simulink model "ofdm_rx"  (R2023b)
settings: Solver=VariableStepAuto  StartTime=0.0  StopTime=10.0  RelTol=1e-3
values from neighbouring files (symbols this model uses):
  Fs = 1e6    (= 1000000)    [offline_analyze_rx_raw.m]    (also in parameter.m)
  payloadIdx = randi([0 M-1], numDataSC*(numOFDMSym-1), 1)    [offline_analyze_rx_demod.m]    (also in parameter.m = randi([0 M-1], numDataSC*numPayloadSym, 1); sim_ofdm_complex.m = randi([0 cfg.M-1], numDataSC*cfg.numPayloadSym, 1))
undefined symbols (not defined in the file or in its folder): ip
libraries: plutoradiolib x1, commsink2 x1, commofdm x1, commdigbbndpm3 x1
settings Model: Creator=yuezh  LastModifiedBy=123

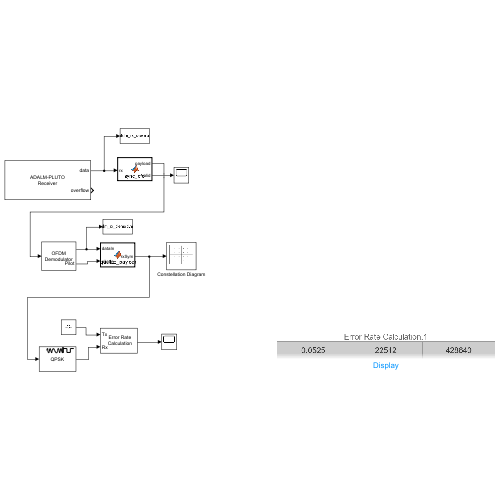
[thumbnail: Simulink's stored preview of the top-level diagram]
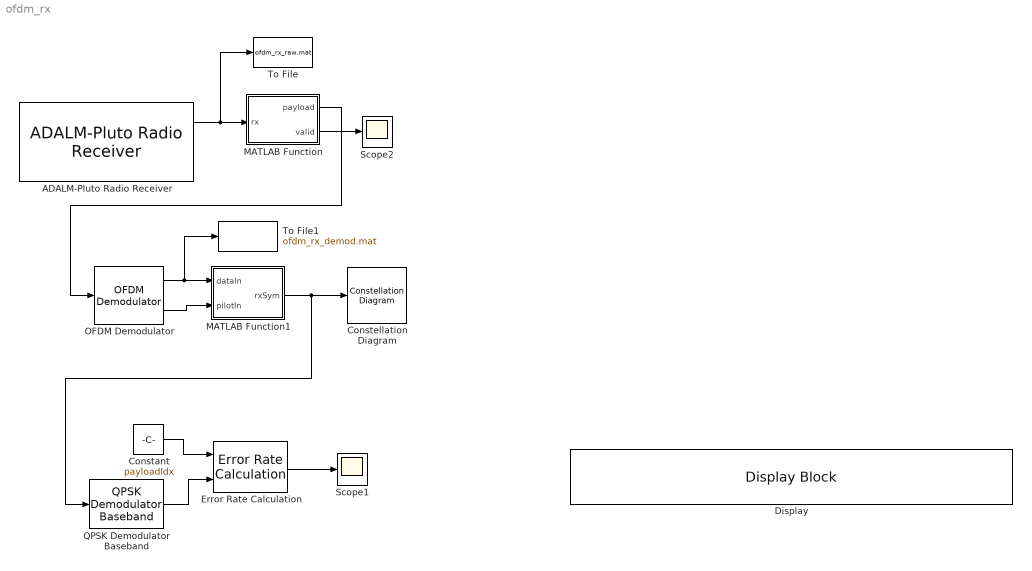
== system ofdm_rx ==
  ADALM-Pluto Radio Receiver : plutoradiolib/ADALM-Pluto Radio Receiver  RadioID=ip:192.168.1.10  uri=ip:10.0.0.200  CenterFrequencySource=Dialog  CenterFrequency=Fc  GainSource=AGC Slow Attack  GainSourceBlock=Dialog  Gain=35  ChannelMapping=1  BasebandSampleRate=Fs  OutputDataType=single  SamplesPerFrame=10080  OverflowOutputPort=on  EnableBurstMode=off  NumFramesInBurst=1  ShowAdvancedProperties=off  UseCustomFilter=off  filtPathRates=[737280000 11520000 3840000 1920000 960000 240000]  filtCoefficients=[-192 82 85 -215 228 -102 -110 290 -318 145 160 -426 471 -215 -238 633 -697 318 349 -923 1009 -457 -498 1309 -1423 640 693 -1812 1959 -876 -945 2458 -2647 1180 1268 -3290 3534 -1572 -1688 4375 -4698 2091 2247 -5836 6284 -2807 -3031 7918 -8588 3870 4225 -11182 12324 -5662 -6330 17255 -19735 9507 11312 -33568 43355 -25227 -42139 305542 305542 -42139 -25227 43355 -33568 11312 9507 -19735 17255 -6330 -5662 12324 -11182 4225 3870 -8588 7918 -3031 -2807 6284 -5836 2247 2091 -4698 4375 -1688 -1572 3534 -3290 1268 1180 -2647 2458 -945 -876 1959 -1812 693 640 -1423 1309 -498 -457 1009 -923 349 318 -697 633 -238 -215 471 -426 160 145 -318 290 -110 -102 228 -215 85 82 -192]  filtCoefficientSize=128  filtDecimInterpFactor=4  filtGain=-12  filtRFBandwidth=18000000  filterConfigStruct=struct()  EnableQuadratureCorrection=on  EnableRFDCCorrection=on  EnableBasebandDCCorrection=on  FrequencyCorrection=0  OverrideSampleTime=off  SampleTime=0.02  DataTimeout=Inf  ENSMPinControlMode=None  BISTLoopbackMode=Disabled  BISTToneInject=Disabled  BISTSignalGen=PRBS  BISTToneFreq=Fs/32  BISTToneLevel=0
  Constant : Constant  Value=payloadIdx  SampleTime=0.01008
  Constellation Diagram : ConstellationDiagram  WindowPosition=[420.000000,142.000000,600.000000,600.000000,]  Visible=on  ScopeFrameLocation=window
  Display : DisplayBlock  Transparency=1
  Error Rate Calculation : commsink2/Error Rate Calculation  N=0  st_delay=0  cp_mode=Entire frame  subframe=[]  PMode=Port  WsName=ErrorVec  RsMode2=off  stop=off  numErr=100  maxBits=1e6
  MATLAB Function : MATLAB Function  TreatAsAtomicUnit=on
  MATLAB Function1 : MATLAB Function  TreatAsAtomicUnit=on
  OFDM Demodulator : commofdm/OFDM Demodulator  StatePerturbationForJacobian=1.0e-05  FFTLength=64  NumGuardBandCarriers=[6; 5]  RemoveDCCarrier=on  PilotOutputPort=on  PilotCarrierIndices=[12; 26; 40; 54]  CyclicPrefixLength=16  OversamplingFactor=1  NumSymbols=11  NumReceiveAntennas=1  SimulateUsing=Interpreted execution
  QPSK Demodulator Baseband : commdigbbndpm3/QPSK Demodulator Baseband  OutType=Integer  DecType=Hard decision  VarSource=Dialog  Variance=1  Dec=Gray  Ph=pi/4  outDtype1=Inherit via internal rule  outDtype2=Inherit via internal rule  derotateFactorWordLen=16  derotateFactorDataTypeStr=Inherit: Same word length as input  derotateFactorLastDataTypeStr=Inherit: Same word length as input
  Scope1 : Scope
  Scope2 : Scope
  To File : ToFile  Filename=ofdm_rx_raw.mat  SaveFormat=Timeseries
  To File1 : ToFile  Filename=ofdm_rx_demod.mat  SaveFormat=Timeseries
  wires:
  ADALM-Pluto Radio Receiver/1 -> To File/1, MATLAB Function/1(rx)
  MATLAB Function/1(payload) -> OFDM Demodulator/1
  MATLAB Function1/1(rxSym) -> Constellation Diagram/1, QPSK Demodulator Baseband/1
  Constant/1 -> Error Rate Calculation/1
  QPSK Demodulator Baseband/1 -> Error Rate Calculation/2
  OFDM Demodulator/1 -> To File1/1, MATLAB Function1/1(dataIn)
  OFDM Demodulator/2 -> MATLAB Function1/2(pilotIn)
  Error Rate Calculation/1 -> Scope1/1
  MATLAB Function/2(valid) -> Scope2/1

== matlab function ofdm_rx/MATLAB Function ==
  data: rx input; payload output; valid output
function [payload, valid] = sync_cfo(rx)
%#codegen

Nfft = 64;
cpLen = 16;
numOFDMSym = 11;
ofdmLen = numOFDMSym * (Nfft + cpLen);

payload = complex(zeros(ofdmLen,1,'single'));
valid = false;

preHalf = exp(1j*2*pi*(0:63).'/8);
preamble = [preHalf; preHalf];

rx = rx(:);
L = length(rx);

if L < length(preamble) + ofdmLen
    return;
end

bestMetric = single(0);
bestIdx = 1;

for k = 1:(L - length(preamble) - ofdmLen + 1)
    seg = rx(k:k+127);
    metric = abs(sum(conj(single(preamble)) .* seg)) / ...
        (sqrt(sum(abs(seg).^2)) * sqrt(sum(abs(single(preamble)).^2)) + eps('single'));
    if metric > bestMetric
        bestMetric = metric;
        bestIdx = k;
    end
end

if bestMetric < 0.45
    return;
end

r1 = rx(bestIdx:bestIdx+63);
r2 = rx(bestIdx+64:bestIdx+127);

phi = angle(sum(conj(r1).*r2));
cfoNorm = phi / (2*pi*Nfft);

startIdx = bestIdx + 128;
x = rx(startIdx:startIdx+ofdmLen-1);

n = single((0:ofdmLen-1).');
payload = x .* exp(-1j*2*pi*single(cfoNorm)*n);

valid = true;

== matlab function ofdm_rx/MATLAB Function1 ==
  data: dataIn input; rxSym output; pilotIn input
function rxSym = equalize_payload(dataIn, pilotIn)
%#codegen

M = 4;
numDataSC = 48;
numPayloadSym = 10;

rng(2);
trainIdx = randi([0 M-1], numDataSC, 1);
trainSym = pskmod(trainIdx, M, pi/4, 'gray');

H = dataIn(:,1) ./ trainSym;
Y = dataIn(:,2:end) ./ H;

Hpilot = pilotIn(:,1);

for k = 1:numPayloadSym
    cpe = mean(pilotIn(:,k+1) ./ Hpilot);
    if abs(cpe) > 0
        Y(:,k) = Y(:,k) ./ (cpe / abs(cpe));
    end
end

rxSym = double(Y(:));
